simulink model "mmc_7"  (R2026a)
settings: Solver=ode14x  StopTime=0.3  FixedStep=1e-6
model workspace (MAT data in the model file):
  N = 8
  Rarm = 1
  Vdc = 40
values from neighbouring files (symbols this model uses):
  C_sm = 220e-6    (= 0.00022)    [parameters.m]
  L_arm = 40e-3    (= 0.04)    [parameters.m]
  lambda_cap = 0.1    [parameters.m]
  lambda_circ = 0.3    [parameters.m]
  lambda_i = 1    [parameters.m]
  lambda_sw = 0.1    [parameters.m]
  P_rated = 1e3    (= 1000)    [parameters.m]
  R_arm = 1208e-3    (= 1.208)    [parameters.m]
  T_sample = 50e-6    (= 5e-05)    [parameters.m]
  V_dc = 750    [parameters.m]
  Vc_nom = V_dc /N    (= 93.75)    [parameters.m]
undefined symbols (not defined in the file or in its folder): cosphi, I_DEADBAND, L_load, m, R_load, V_TOL
libraries: nesl_utility x155, fl_lib x111, ee_lib x107
(part 14 of 14)

== matlab function mmc_7/Subsystem5/MATLAB Function2 ==
  data: Gate1u output; Gate2u output; Gate1l output; Gate2l output; vcu input; Su output size=[8 1]; vcl input; nu input; nl input; i_upper input; i_lower input; Su_prev input; Sl_prev input; Sl output size=[8 1]; N input; I_DEADBAND input; V_TOL input
function [Gate1u, Gate2u, Gate1l, Gate2l, Su, Sl] = Voltage_Sorting( ...
    vcu, vcl, nu, nl, i_upper, i_lower, Su_prev, Sl_prev, N , I_DEADBAND, V_TOL) 
%VOLTAGE_SORTING  Sort-and-select balancing for one MMC phase leg, N=8
% half-bridge submodules per arm. 
% Outputs the two complementary gate signals each half-bridge SM physically requires.
%
% INPUTS
%   vcu, vcl        - [1xN] upper/lower arm submodule capacitor voltages [V]
%   nu, nl          - required insertion counts
%   i_upper,i_lower - measured arm currents (sign decides charge/discharge)
%   Su_prev,Sl_prev - [1xN] previous cycle's insertion states (hysteresis
%                     input, fed back externally via Unit Delay)
%   N               - submodules per arm (compile-time constant, = 8)
%
% OUTPUTS
%   Gate1u,Gate2u   - [1xN] upper arm gate pairs (Gate2 = NOT(Gate1))
%   Gate1l,Gate2l   - [1xN] lower arm gate pairs
%   Su, Sl          - [1xN] insertion states this cycle (1=insert,0=bypass) --
%                     feed back externally via Unit Delay as next cycle's
%                     Su_prev/Sl_prev


Su = zeros(N,1);
Sl = zeros(N,1);
Gate1u = zeros(N,1);
Gate1l = zeros(N,1);
Gate2u = zeros(N,1);
Gate2l = zeros(N,1);

Su = select_one_arm(vcu, nu, i_upper, Su_prev, N, I_DEADBAND, V_TOL);
Sl = select_one_arm(vcl, nl, i_lower, Sl_prev, N, I_DEADBAND, V_TOL);

Gate1u = Su;              Gate2u = double(~Su);
Gate1l = Sl;              Gate2l = double(~Sl);
end

function S = select_one_arm(vc, n_ins, i_arm, S_prev, N, I_DEADBAND, V_TOL)
S = zeros(N,1);
[~, idx_ascend] = sort(vc, 'ascend');   % idx_ascend(1) = lowest-voltage SM

if i_arm > I_DEADBAND
    idx_sel = idx_ascend;                 % charging: lowest-V first
elseif i_arm < -I_DEADBAND
    idx_sel = idx_ascend(N:-1:1);         % discharging: highest-V first
else
    % Deadband: pick whichever direction needs fewer state changes
    cand_charge    = zeros(N,1); 
    cand_discharge = zeros(N,1); 


    for m = 1:N
        if m <= n_ins
            cand_charge(idx_ascend(m)) = 1;
            cand_discharge(idx_ascend(N - n_ins + m)) = 1;
        end
    end

    if sum(abs(cand_charge - S_prev)) <= sum(abs(cand_discharge - S_prev))
        idx_sel = idx_ascend;
    else
        idx_sel = idx_ascend(N:-1:1);
    end
end


for m = 1:N
    if m <= n_ins
        S(idx_sel(m)) = 1;
    end
end

% Hysteresis pass: 
for j = 1:N
    if S(j) ~= S_prev(j)
        for k = 1:N
            if k ~= j && S(k)==S_prev(j) && S_prev(k)==S(j) ...
                    && abs(vc(j)-vc(k)) < V_TOL
                tmp = S(j); S(j) = S(k); S(k) = tmp;
            end
        end
    end
end
end

== matlab function mmc_7/Subsystem/MATLAB Function1 ==
  data: i_ref input; nu_opt output; i_out_meas input; i_circ_meas input; i_upper input; i_lower input; vcu input; vcl input; Vdc input; Ts input; Csm input; nu_prev input; nl_prev input; Larm input; Rarm input; L_load input; R_load input; lambda_i input; lambda_sw input; lambda_cap input; lambda_circ input; nl_opt output; J_opt output; cand_idx output; dbg output; P_rated input; m input; cos_phi input; N input; Vc_nom input
function [nu_opt, nl_opt, J_opt, cand_idx,dbg] = Indirect_FCS_MPC( ...
    i_ref, i_out_meas, i_circ_meas,...
i_upper, i_lower, ...
    vcu, vcl, Vdc, Ts, Csm, ...
    nu_prev, nl_prev, ...
    Larm, Rarm, L_load, R_load, ...
    lambda_i, lambda_sw, lambda_cap, lambda_circ,...
    P_rated,m,cos_phi,N, Vc_nom) 

%INDIRECT_FCS_MPC Per-phase MPC: Relaxed search over insertion
% COUNTS (nu,nl), evaluating safe candidates for N=8.

% INPUTS
% i_ref - reference output (load) current, this phase [A]
% i_out_meas - measured output/load current, this phase [A]
% i_circ_meas - measured circulating current, this phase [A]
% i_upper - measured upper arm current [A]
% i_lower - measured lower arm current [A]
% vcu - [1xN] upper arm submodule capacitor voltages [V]
% vcl - [1xN] lower arm submodule capacitor voltages [V]
% Vdc - DC link voltage [V]
% Ts - sample time [s]
% N - submodules per arm (compile-time constant, e.g. 8)
% Csm - submodule capacitance [F]
% nu_prev,nl_prev - previous cycle's chosen insertion counts (real
% fed-back state, not re-estimated from a measurement)
% Larm, Rarm - arm inductance , arm resistance
% L_load,R_load - load inductance / load resistance
% lambda_* - cost function weights
% P_rated, m, cosphi - Operating parameters for I_max dynamic calculation
% Vc_nom - nominal capacitor voltage

% OUTPUTS
% nu_opt, nl_opt - chosen upper/lower insertion counts
% J_opt - cost of the chosen candidate
% cand_idx - linear candidate index, nu_opt*(N+1)+nl_opt+1 (1..81)
% -- useful as a direct classification label for later
% ML-surrogate training data
% dbg - [io_pred_opt,icirc_pred_opt, vcu_avg_pred_opt,vcl_avg_pred_opt]

%% Step 0 - aggregate measured quantities and effective circuit params
vcu_avg = mean(vcu);
vcl_avg = mean(vcl);
L_eff = L_load + Larm/2;
R_eff = R_load + Rarm/2;
icirc_ref = 0; % standard suppression target

% ADDED: Maximum Current Limit (I_max) Calculation 
I_dc = P_rated / Vdc; 
I_arm_dc = I_dc / 3;

V_s_peak = m * Vdc / 2;
I_s_peak = (4 * P_rated) / (3 * m * Vdc * cos_phi);
I_arm_ac = I_s_peak / 2;

I_max = I_arm_ac + I_arm_dc;

%% Step 1 - Relaxed exhaustive search bounded by constraints
J_best = 1e12;
% Fail-safe: Initialize to previous state so if a transient causes all 
% candidates to violate I_max, the converter holds its state instead of shorting (0,0)
nu_opt = nu_prev; 
nl_opt = nl_prev; 

io_pred_opt = i_out_meas;
icirc_pred_opt = i_circ_meas;
vcu_avg_pred_opt = vcu_avg;
vcl_avg_pred_opt = vcl_avg;
for nu = 0:N
    for nl = 0:N

        % Relaxed Constraint Boundary 
        sum_ins = nu + nl;
        if sum_ins >= (N - 1) && sum_ins <= (N + 1)

            vconv_c = (nl*vcl_avg - nu*vcu_avg) / 2;
            vcommon_c = (nu*vcu_avg + nl*vcl_avg) / 2;

            io_pred = i_out_meas + (Ts/L_eff)*(vconv_c - R_eff*i_out_meas);
            icirc_pred = i_circ_meas + (Ts/Larm)*(Vdc/2 - vcommon_c - Rarm*i_circ_meas);

            % Calculate what the arm currents will be based on predictions
            i_upper_pred = (io_pred / 2) + icirc_pred;
            i_lower_pred = -(io_pred / 2) + icirc_pred;

            % If either predicted arm current exceeds the calculated limit, discard state
            if abs(i_upper_pred) > I_max || abs(i_lower_pred) > I_max
                continue; 
            end
            

            vcu_avg_pred = vcu_avg + (Ts*nu/(N*Csm))*i_upper;
            vcl_avg_pred = vcl_avg + (Ts*nl/(N*Csm))*i_lower;

            J_current = (i_ref - io_pred)^2;
            J_switch = (nu-nu_prev)^2 + (nl-nl_prev)^2;
            J_cap = ((vcu_avg_pred^2 - vcl_avg_pred^2)/(2*Vc_nom^2))^2;
            J_circ = (icirc_ref - icirc_pred)^2;

            J_total = lambda_i*J_current + lambda_sw*J_switch + lambda_cap*J_cap + lambda_circ*J_circ;

            if J_total < J_best
                J_best = J_total;
                nu_opt = nu; nl_opt = nl;
                io_pred_opt = io_pred;
                icirc_pred_opt = icirc_pred;
                vcu_avg_pred_opt = vcu_avg_pred; 
                vcl_avg_pred_opt = vcl_avg_pred;
            end

        end
    end
end

J_opt = J_best;
cand_idx = nu_opt*(N+1) + nl_opt + 1; % deterministic label
dbg = [io_pred_opt, icirc_pred_opt, vcu_avg_pred_opt, vcl_avg_pred_opt];

end

== matlab function mmc_7/Subsystem/MATLAB Function2 ==
  data: Gate1u output; Gate2u output; Gate1l output; Gate2l output; vcu input; Su output size=[8 1]; vcl input; nu input; nl input; i_upper input; i_lower input; Su_prev input; Sl_prev input; Sl output size=[8 1]; N input; I_DEADBAND input; V_TOL input
function [Gate1u, Gate2u, Gate1l, Gate2l, Su, Sl] = Voltage_Sorting( ...
    vcu, vcl, nu, nl, i_upper, i_lower, Su_prev, Sl_prev, N , I_DEADBAND, V_TOL) 
%VOLTAGE_SORTING  Sort-and-select balancing for one MMC phase leg, N=8
% half-bridge submodules per arm. 
% Outputs the two complementary gate signals each half-bridge SM physically requires.
%
% INPUTS
%   vcu, vcl        - [1xN] upper/lower arm submodule capacitor voltages [V]
%   nu, nl          - required insertion counts
%   i_upper,i_lower - measured arm currents (sign decides charge/discharge)
%   Su_prev,Sl_prev - [1xN] previous cycle's insertion states (hysteresis
%                     input, fed back externally via Unit Delay)
%   N               - submodules per arm (compile-time constant, = 8)
%
% OUTPUTS
%   Gate1u,Gate2u   - [1xN] upper arm gate pairs (Gate2 = NOT(Gate1))
%   Gate1l,Gate2l   - [1xN] lower arm gate pairs
%   Su, Sl          - [1xN] insertion states this cycle (1=insert,0=bypass) --
%                     feed back externally via Unit Delay as next cycle's
%                     Su_prev/Sl_prev


Su = zeros(N,1);
Sl = zeros(N,1);
Gate1u = zeros(N,1);
Gate1l = zeros(N,1);
Gate2u = zeros(N,1);
Gate2l = zeros(N,1);

Su = select_one_arm(vcu, nu, i_upper, Su_prev, N, I_DEADBAND, V_TOL);
Sl = select_one_arm(vcl, nl, i_lower, Sl_prev, N, I_DEADBAND, V_TOL);

Gate1u = Su;              Gate2u = double(~Su);
Gate1l = Sl;              Gate2l = double(~Sl);
end

function S = select_one_arm(vc, n_ins, i_arm, S_prev, N, I_DEADBAND, V_TOL)
S = zeros(N,1);
[~, idx_ascend] = sort(vc, 'ascend');   % idx_ascend(1) = lowest-voltage SM

if i_arm > I_DEADBAND
    idx_sel = idx_ascend;                 % charging: lowest-V first
elseif i_arm < -I_DEADBAND
    idx_sel = idx_ascend(N:-1:1);         % discharging: highest-V first
else
    % Deadband: pick whichever direction needs fewer state changes
    cand_charge    = zeros(N,1); 
    cand_discharge = zeros(N,1); 


    for m = 1:N
        if m <= n_ins
            cand_charge(idx_ascend(m)) = 1;
            cand_discharge(idx_ascend(N - n_ins + m)) = 1;
        end
    end

    if sum(abs(cand_charge - S_prev)) <= sum(abs(cand_discharge - S_prev))
        idx_sel = idx_ascend;
    else
        idx_sel = idx_ascend(N:-1:1);
    end
end


for m = 1:N
    if m <= n_ins
        S(idx_sel(m)) = 1;
    end
end

% Hysteresis pass: 
for j = 1:N
    if S(j) ~= S_prev(j)
        for k = 1:N
            if k ~= j && S(k)==S_prev(j) && S_prev(k)==S(j) ...
                    && abs(vc(j)-vc(k)) < V_TOL
                tmp = S(j); S(j) = S(k); S(k) = tmp;
            end
        end
    end
end
end

== matlab function mmc_7/Subsystem4/MATLAB Function1 ==
  data: i_ref input; nu_opt output; i_out_meas input; i_circ_meas input; i_upper input; i_lower input; vcu input; vcl input; Vdc input; Ts input; Csm input; nu_prev input; nl_prev input; Larm input; Rarm input; L_load input; R_load input; lambda_i input; lambda_sw input; lambda_cap input; lambda_circ input; nl_opt output; J_opt output; cand_idx output; dbg output; P_rated input; m input; cos_phi input; N input; Vc_nom input
function [nu_opt, nl_opt, J_opt, cand_idx,dbg] = Indirect_FCS_MPC( ...
    i_ref, i_out_meas, i_circ_meas,...
i_upper, i_lower, ...
    vcu, vcl, Vdc, Ts, Csm, ...
    nu_prev, nl_prev, ...
    Larm, Rarm, L_load, R_load, ...
    lambda_i, lambda_sw, lambda_cap, lambda_circ,...
    P_rated,m,cos_phi,N, Vc_nom) 

%INDIRECT_FCS_MPC Per-phase MPC: Relaxed search over insertion
% COUNTS (nu,nl), evaluating safe candidates for N=8.

% INPUTS
% i_ref - reference output (load) current, this phase [A]
% i_out_meas - measured output/load current, this phase [A]
% i_circ_meas - measured circulating current, this phase [A]
% i_upper - measured upper arm current [A]
% i_lower - measured lower arm current [A]
% vcu - [1xN] upper arm submodule capacitor voltages [V]
% vcl - [1xN] lower arm submodule capacitor voltages [V]
% Vdc - DC link voltage [V]
% Ts - sample time [s]
% N - submodules per arm (compile-time constant, e.g. 8)
% Csm - submodule capacitance [F]
% nu_prev,nl_prev - previous cycle's chosen insertion counts (real
% fed-back state, not re-estimated from a measurement)
% Larm, Rarm - arm inductance , arm resistance
% L_load,R_load - load inductance / load resistance
% lambda_* - cost function weights
% P_rated, m, cosphi - Operating parameters for I_max dynamic calculation
% Vc_nom - nominal capacitor voltage

% OUTPUTS
% nu_opt, nl_opt - chosen upper/lower insertion counts
% J_opt - cost of the chosen candidate
% cand_idx - linear candidate index, nu_opt*(N+1)+nl_opt+1 (1..81)
% -- useful as a direct classification label for later
% ML-surrogate training data
% dbg - [io_pred_opt,icirc_pred_opt, vcu_avg_pred_opt,vcl_avg_pred_opt]

%% Step 0 - aggregate measured quantities and effective circuit params
vcu_avg = mean(vcu);
vcl_avg = mean(vcl);
L_eff = L_load + Larm/2;
R_eff = R_load + Rarm/2;
icirc_ref = 0; % standard suppression target

% ADDED: Maximum Current Limit (I_max) Calculation 
I_dc = P_rated / Vdc; 
I_arm_dc = I_dc / 3;

V_s_peak = m * Vdc / 2;
I_s_peak = (4 * P_rated) / (3 * m * Vdc * cos_phi);
I_arm_ac = I_s_peak / 2;

I_max = I_arm_ac + I_arm_dc;

%% Step 1 - Relaxed exhaustive search bounded by constraints
J_best = 1e12;
% Fail-safe: Initialize to previous state so if a transient causes all 
% candidates to violate I_max, the converter holds its state instead of shorting (0,0)
nu_opt = nu_prev; 
nl_opt = nl_prev; 

io_pred_opt = i_out_meas;
icirc_pred_opt = i_circ_meas;
vcu_avg_pred_opt = vcu_avg;
vcl_avg_pred_opt = vcl_avg;
for nu = 0:N
    for nl = 0:N

        % Relaxed Constraint Boundary 
        sum_ins = nu + nl;
        if sum_ins >= (N - 1) && sum_ins <= (N + 1)

            vconv_c = (nl*vcl_avg - nu*vcu_avg) / 2;
            vcommon_c = (nu*vcu_avg + nl*vcl_avg) / 2;

            io_pred = i_out_meas + (Ts/L_eff)*(vconv_c - R_eff*i_out_meas);
            icirc_pred = i_circ_meas + (Ts/Larm)*(Vdc/2 - vcommon_c - Rarm*i_circ_meas);

            % Calculate what the arm currents will be based on predictions
            i_upper_pred = (io_pred / 2) + icirc_pred;
            i_lower_pred = -(io_pred / 2) + icirc_pred;

            % If either predicted arm current exceeds the calculated limit, discard state
            if abs(i_upper_pred) > I_max || abs(i_lower_pred) > I_max
                continue; 
            end
            

            vcu_avg_pred = vcu_avg + (Ts*nu/(N*Csm))*i_upper;
            vcl_avg_pred = vcl_avg + (Ts*nl/(N*Csm))*i_lower;

            J_current = (i_ref - io_pred)^2;
            J_switch = (nu-nu_prev)^2 + (nl-nl_prev)^2;
            J_cap = ((vcu_avg_pred^2 - vcl_avg_pred^2)/(2*Vc_nom^2))^2;
            J_circ = (icirc_ref - icirc_pred)^2;

            J_total = lambda_i*J_current + lambda_sw*J_switch + lambda_cap*J_cap + lambda_circ*J_circ;

            if J_total < J_best
                J_best = J_total;
                nu_opt = nu; nl_opt = nl;
                io_pred_opt = io_pred;
                icirc_pred_opt = icirc_pred;
                vcu_avg_pred_opt = vcu_avg_pred; 
                vcl_avg_pred_opt = vcl_avg_pred;
            end

        end
    end
end

J_opt = J_best;
cand_idx = nu_opt*(N+1) + nl_opt + 1; % deterministic label
dbg = [io_pred_opt, icirc_pred_opt, vcu_avg_pred_opt, vcl_avg_pred_opt];

end
